simulink model "septum"  (R2024b)
settings: Solver=VariableStepAuto  StartTime=0.0  StopTime=4  RelTol=1e-3
InitFcn:
  | Tint = 1e-6
  | Ts = 100*Tint
libraries: spsIGBTDiodeLib x6, spsSeriesRLCBranchLib x5, spsCurrentMeasurementLib x4, spsVoltageMeasurementLib x4, simulink x2, spsGroundLib x1, spsPowerPositiveSequenceLib x1, spsThreePhaseVIMeasurementLib x1, spsThreePhaseSourceLib x1, spspowerguiLib x1
settings Model: Creator=dagua  LastModifiedBy=dagua
settings DataIOCC: ReturnWorkspaceOutputs=off

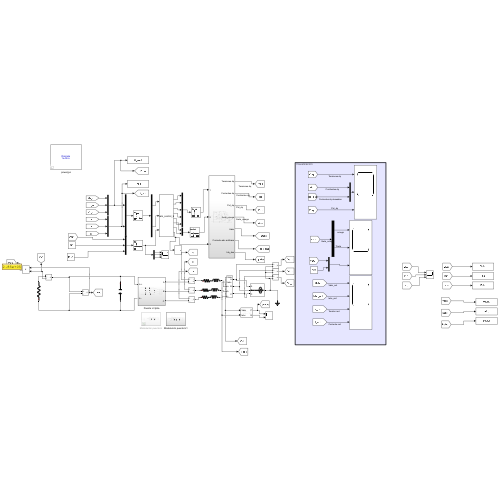
[thumbnail: Simulink's stored preview of the top-level diagram]
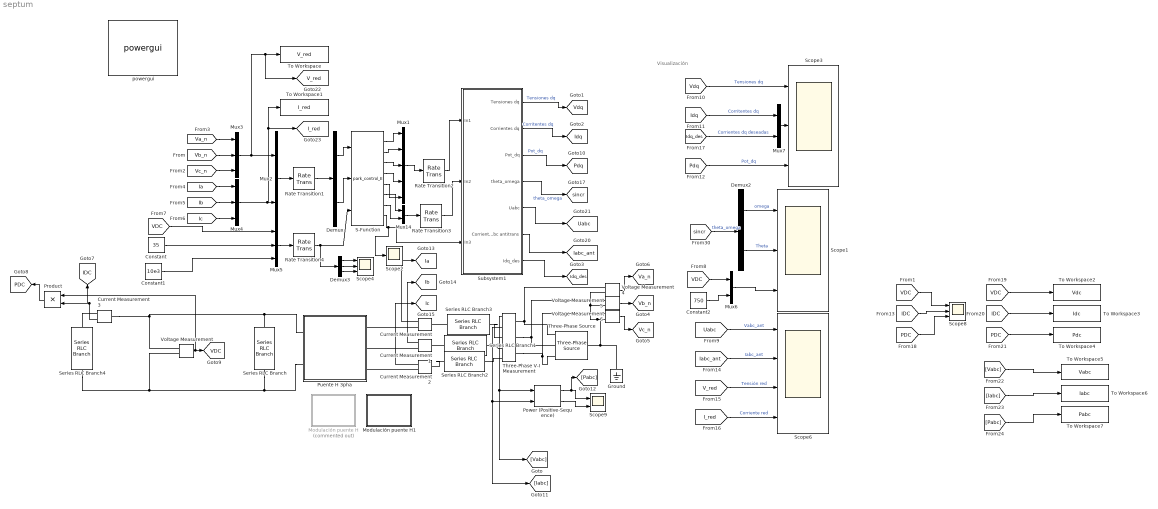
== system septum ==
  note: Visualización
  Constant : Constant  Value=35
  Constant1 : Constant  Value=10e3
  Constant2 : Constant  Value=750
  Current Measurement{,1..3} (4 alike) : spsCurrentMeasurementLib/Current Measurement  PhasorSimulation=off  OutputType=Complex  PSBequivalent=0
  Demux : Demux  Outputs=2
  Demux2 : Demux  Outputs=2
  Demux3 : Demux  Outputs=3
  Ground : spsGroundLib/Ground  LConnTagsString=a
  Modulación puente H : Subsystem  Commented=on
  Modulación puente H1 : Subsystem
  Mux1 : Mux  Inputs=5
  Mux{2,6..7,14} (4 alike) : Mux  Inputs=2
  Mux3 : Mux  Inputs=3
  Mux4 : Mux  Inputs=3
  Mux5 : Mux  Inputs=3
  Power (Positive-Sequence) : spsPowerPositiveSequenceLib/Power (Positive-Sequence)  Freq=50  Vinit=[0, 0]  Iinit=[0, 0]  Ts=0
      settings: LibrarySourceBlock=|
      | sps_lib/Sensors and Measurements/Power
      | (Positive-Sequence)
  Product : Product
  Puente H 3pha : Subsystem
  Rate Transition1 : RateTransition  OutPortSampleTime=Ts
  Rate Transition2 : RateTransition  Deterministic=off  InitialCondition=[0]  OutPortSampleTime=Tint
  Rate Transition3 : RateTransition  Deterministic=off  InitialCondition=[0]  OutPortSampleTime=Tint
  Rate Transition4 : RateTransition  OutPortSampleTime=Ts
  S-Function : S-Function  FunctionName=park_control_E  SFunctionDeploymentMode=off  EnableBusSupport=off
  Scope{1,3..4,8} (4 alike) : Scope  NumInputPorts=3
  Scope2 : Scope
  Scope6 : Scope  NumInputPorts=4
  Scope9 : Scope  NumInputPorts=2
  Series RLC Branch : spsSeriesRLCBranchLib/Series RLC Branch  LConnTagsString=__new0  RConnTagsString=__new0  BranchType=C  Resistance=1  Inductance=1e-3  SetiL0=off  InitialCurrent=0  Capacitance=3300e-4  Setx0=on  InitialVoltage=10  Measurements=None
  Series RLC Branch1 : spsSeriesRLCBranchLib/Series RLC Branch  LConnTagsString=__new0  RConnTagsString=__new0  BranchType=RL  Resistance=0.01  Inductance=12e-5  SetiL0=off  InitialCurrent=0  Capacitance=1e-6  Setx0=off  InitialVoltage=0  Measurements=None
  Series RLC Branch2 : spsSeriesRLCBranchLib/Series RLC Branch  LConnTagsString=__new0  RConnTagsString=__new0  BranchType=RL  Resistance=0.01  Inductance=12e-5  SetiL0=off  InitialCurrent=0  Capacitance=1e-6  Setx0=off  InitialVoltage=0  Measurements=None
  Series RLC Branch3 : spsSeriesRLCBranchLib/Series RLC Branch  LConnTagsString=__new0  RConnTagsString=__new0  BranchType=RL  Resistance=0.01  Inductance=12e-5  SetiL0=off  InitialCurrent=0  Capacitance=1e-6  Setx0=off  InitialVoltage=0  Measurements=None
  Series RLC Branch4 : spsSeriesRLCBranchLib/Series RLC Branch  LConnTagsString=__new0  RConnTagsString=__new0  BranchType=R  Resistance=35*35/267.47e3  Inductance=1e-3  SetiL0=off  InitialCurrent=0  Capacitance=1e-6  Setx0=off  InitialVoltage=0  Measurements=None
  Subsystem1 : Subsystem
  Three-Phase V-I Measurement : spsThreePhaseVIMeasurementLib/Three-Phase V-I Measurement  VoltageMeasurement=phase-to-ground  SetLabelV=off  LabelV=Vabc  Vpu=off  VpuLL=off  CurrentMeasurement=yes  SetLabelI=off  LabelI=Iabc  Ipu=off  Pbase=100e6  Vbase=500e3  OutputType=Complex  PhasorSimulation=off  PSBequivalent=0
  Three-Phase Source : spsThreePhaseSourceLib/Three-Phase Source  InternalConnection=Yn  VoltagePhases=off  Voltage=400  PhaseAngle=0  Voltage_phases=[25e3 25e3 25e3]/sqrt(3)  PhaseAngles_phases=[0 -120 +120]  Frequency=50  NonIdealSource=off  SpecifyImpedance=off  Resistance=0.8929  Inductance=16.58e-3  ShortCircuitLevel=100e6  BaseVoltage=25e3  XRratio=7  BusType=PV  Pref=400e3  Qref=0  Prefabc=[10e3, 10e3, 10e3]  Qrefabc=[0, 0, 0]  Qmin=-inf  Qmax=inf
  To Workspace : ToWorkspace  VariableName=V_red  SaveFormat=Timeseries  SampleTime=-1
  To Workspace1 : ToWorkspace  VariableName=I_red  SaveFormat=Timeseries  SampleTime=-1
  To Workspace2 : ToWorkspace  VariableName=Vdc  SaveFormat=Timeseries  SampleTime=-1
  To Workspace3 : ToWorkspace  VariableName=Idc  SaveFormat=Timeseries  SampleTime=-1
  To Workspace4 : ToWorkspace  VariableName=Pdc  SaveFormat=Timeseries  SampleTime=-1
  To Workspace5 : ToWorkspace  VariableName=Vabc  SaveFormat=Timeseries  SampleTime=-1
  To Workspace6 : ToWorkspace  VariableName=Iabc  SaveFormat=Timeseries  SampleTime=-1
  To Workspace7 : ToWorkspace  VariableName=Pabc  SaveFormat=Timeseries  SampleTime=-1
  Voltage Measurement{,4..6} (4 alike) : spsVoltageMeasurementLib/Voltage Measurement  PhasorSimulation=off  OutputType=Complex  PSBequivalent=0
  powergui : spspowerguiLib/powergui  Priority=1  SimulationMode=Discrete  SampleTime=Tint  frequency=60  Iterations=50  frequencyindice=0  Pbase=100e6  ErrMax=1e-4  UnitsV=kV  UnitsW=MW  buscounter=0  FunctionMessages=off  echomessages=off  EnableUseOfTLC=off  CurrentSourceSwitches=off  DisableSnubberDevices=off  DisableRonSwitches=off  DisableVfSwitches=off  DisplayEquations=off  AutomaticDiscreteSolvers=off  SolverType=Tustin  Interpol=off  ExternalGateDelay=off  methode=off  Ts=0  x0status=blocks  SPID=off  SwTol=0  HookPort=off  NonlinearTolerance=1e-4  nMaxIteration=100  ContinueOnMaxIteration=off  RestoreLinks=warning  ResistiveCurrentMeasurement=off  Frange=[0:2:500]  Ylog=off  Xlog=on  ShowGrid=off  save=off  variable=ZData  structure=Iabc  ZoomFFT=off  StartTime=0.36  cycles=2  DisplayStyle=1  fundamental=50  FreqAxis=off  MaxFrequency=2500  frequencyindicesteady=1  RmsSteady=1  display=off
  tag scope: IDC=global, I_red=global, Ia=global, Iabc_ant=global, Ib=global, Ic=global, Idq=global, Idq_des=global, PDC=global, Pdq=global, Uabc=global, VDC=global, V_red=global, Va_n=global, Vb_n=global, Vc_n=global, Vdq=global, sincr=global
  wires:
  Mux2/1 -> Rate Transition1/1
  S-Function/1 -> Mux1/1
  [Ia] -> Mux4/1
  Rate Transition3/1 -> Subsystem1/2(In2)
  [Ic] -> Mux4/3
  Mux14/1 -> Rate Transition3/1
  Mux3/1 -> [V_red], To Workspace/1, Mux2/1
  Mux5/1 -> Rate Transition4/1
  [V_red] -> Scope6/3  "Tensión red"
  Demux/2 -> S-Function/2
  Demux2/2 -> Scope1/2  "Theta"
  [Pdq] -> Scope3/3  "Pot_dq"
  Subsystem1/7(Idq_des) -> [Idq_des]
  Voltage Measurement/1 -> Product/1, [VDC]
  Current Measurement/1 -> [Ia]
  [VDC] -> Mux6/1
  [Uabc] -> Scope6/1  "Vabc_ant"
  Demux2/1 -> Scope1/1  "omega"
  Demux/1 -> S-Function/1
  [sincr] -> Demux2/1  "theta_omega"
  [Idq] -> Mux7/1  "Corritentes dq"
  [Va_n] -> Mux3/1
  S-Function/6 -> Mux14/1
  Subsystem1/5(Uabc) -> [Uabc]
  S-Function/7 -> Mux14/2
  Subsystem1/1(Tensiones dq) -> [Vdq]  "Tensiones dq"
  Voltage Measurement4/1 -> [Va_n]
  S-Function/5 -> Mux1/5
  [Vdq] -> Scope3/1  "Tensiones dq"
  S-Function/4 -> Mux1/4
  [Ib] -> Mux4/2
  Subsystem1/4(theta_omega) -> [sincr]  "theta_omega"
  Voltage Measurement6/1 -> [Vc_n]
  Subsystem1/2(Corrientes dq) -> [Idq]  "Corritentes dq"
  [Idq_des] -> Mux7/2  "Corrientes dq deseadas"
  [Iabc_ant] -> Scope6/2  "Iabc_ant"
  Rate Transition4/1 -> Demux3/1, S-Function/3
  Mux4/1 -> To Workspace1/1, [I_red], Mux2/2
  Current Measurement2/1 -> [Ic]
  Constant2/1 -> Mux6/2
  Mux1/1 -> Rate Transition2/1
  Subsystem1/6(Corriente abc antitrans) -> [Iabc_ant]
  S-Function/2 -> Mux1/2
  [VDC] -> Mux5/1
  Voltage Measurement5/1 -> [Vb_n]
  S-Function/3 -> Mux1/3
  Rate Transition2/1 -> Subsystem1/1(In1)
  [Vc_n] -> Mux3/3
  [I_red] -> Scope6/4  "Corriente red"
  Current Measurement1/1 -> [Ib]
  Mux7/1 -> Scope3/2
  Constant/1 -> Mux5/2
  Constant1/1 -> Mux5/3
  [Vb_n] -> Mux3/2
  Subsystem1/3(Pot_dq) -> [Pdq]  "Pot_dq"
  Rate Transition1/1 -> Demux/1
  Mux6/1 -> Scope1/3
  Current Measurement3/1 -> [IDC], Product/2
  Product/1 -> [PDC]
  Demux3/1 -> Scope4/1
  Demux3/2 -> Scope4/2
  Demux3/3 -> Scope4/3
  S-Function/8 -> Scope2/1, Subsystem1/3(In3)
  [Pabc] -> To Workspace7/1
  [IDC] -> Scope8/2
  [PDC] -> Scope8/3
  [VDC] -> To Workspace2/1
  [PDC] -> To Workspace4/1
  [VDC] -> Scope8/1
  [Iabc] -> To Workspace6/1
  [IDC] -> To Workspace3/1
  [Vabc] -> To Workspace5/1
  Power (Positive-Sequence)/1 -> [Pabc], Scope9/1
  Power (Positive-Sequence)/2 -> Scope9/2
  Three-Phase V-I Measurement/2 -> [Iabc], Power (Positive-Sequence)/2
  Three-Phase V-I Measurement/1 -> Power (Positive-Sequence)/1, [Vabc]
  connections:
  Voltage Measurement4/LConn2 -- Voltage Measurement5/LConn2 -- Voltage Measurement6/LConn2 -- Three-Phase Source/LConn1 -- Ground/LConn1
  Puente H 3pha/LConn1 -- Current Measurement3/LConn1 -- Voltage Measurement/LConn1 -- Series RLC Branch/LConn1
  Three-Phase Source/RConn3 -- Three-Phase V-I Measurement/LConn3 -- Voltage Measurement6/LConn1
  Puente H 3pha/LConn2 -- Series RLC Branch4/LConn1 -- Voltage Measurement/LConn2 -- Series RLC Branch/RConn1
  Voltage Measurement4/LConn1 -- Three-Phase V-I Measurement/LConn1 -- Three-Phase Source/RConn1
  Three-Phase Source/RConn2 -- Three-Phase V-I Measurement/LConn2 -- Voltage Measurement5/LConn1
  Current Measurement/RConn1 -- Puente H 3pha/RConn1
  Current Measurement2/RConn1 -- Puente H 3pha/RConn3
  Series RLC Branch1/LConn1 -- Current Measurement1/LConn1
  Series RLC Branch2/LConn1 -- Current Measurement2/LConn1
  Series RLC Branch3/LConn1 -- Current Measurement/LConn1
  Current Measurement1/RConn1 -- Puente H 3pha/RConn2
  Series RLC Branch4/RConn1 -- Current Measurement3/RConn1
  Series RLC Branch3/RConn1 -- Three-Phase V-I Measurement/RConn1
  Series RLC Branch1/RConn1 -- Three-Phase V-I Measurement/RConn2
  Series RLC Branch2/RConn1 -- Three-Phase V-I Measurement/RConn3

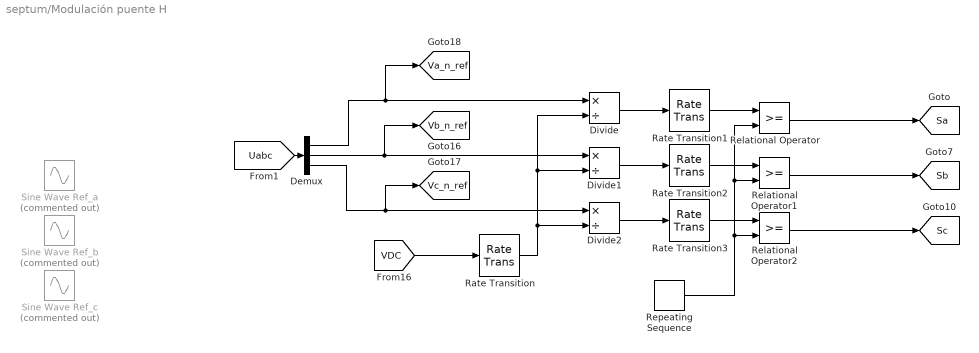
== system septum/Modulación puente H ==
  Demux : Demux  Outputs=3
  Divide : Product  Inputs=*/
  Divide1 : Product  Inputs=*/
  Divide2 : Product  Inputs=*/
  Rate Transition : RateTransition  OutPortSampleTime=Ts
  Rate Transition1 : RateTransition  OutPortSampleTime=Tint
  Rate Transition2 : RateTransition  OutPortSampleTime=Tint
  Rate Transition3 : RateTransition  OutPortSampleTime=Tint
  Relational Operator : RelationalOperator  OutDataTypeStr=boolean  RndMeth=Simplest  InputSameDT=off
  Relational Operator1 : RelationalOperator  OutDataTypeStr=boolean  RndMeth=Simplest  InputSameDT=off
  Relational Operator2 : RelationalOperator  OutDataTypeStr=boolean  RndMeth=Simplest  InputSameDT=off
  Repeating Sequence : simulink/Sources/Repeating Sequence  rep_seq_t=[0 Ts/2 Ts]  rep_seq_y=[-1 1 -1]
  Sine Wave Ref_a : Sin  Commented=on  Amplitude=370  Frequency=2*pi*50  SampleTime=Ts
  Sine Wave Ref_b : Sin  Commented=on  Amplitude=370  Frequency=2*pi*50  Phase=120*2*pi/360  SampleTime=Ts
  Sine Wave Ref_c : Sin  Commented=on  Amplitude=370  Frequency=2*pi*50  Phase=-120*2*pi/360  SampleTime=Ts
  tag scope: Sa=global, Sb=global, Sc=global, Va_n_ref=global, Vb_n_ref=global, Vc_n_ref=global
  wires:
  Demux/3 -> [Vc_n_ref], Divide2/1
  Demux/1 -> Divide/1, [Va_n_ref]
  Demux/2 -> [Vb_n_ref], Divide1/1
  [VDC] -> Rate Transition/1
  Relational Operator/1 -> [Sa]
  Relational Operator1/1 -> [Sb]
  Relational Operator2/1 -> [Sc]
  Rate Transition/1 -> Divide2/2, Divide1/2, Divide/2
  Rate Transition1/1 -> Relational Operator/1
  Divide1/1 -> Rate Transition2/1
  Rate Transition2/1 -> Relational Operator1/1
  Divide2/1 -> Rate Transition3/1
  Rate Transition3/1 -> Relational Operator2/1
  Repeating Sequence/1 -> Relational Operator2/2, Relational Operator1/2, Relational Operator/2
  Divide/1 -> Rate Transition1/1
  [Uabc] -> Demux/1

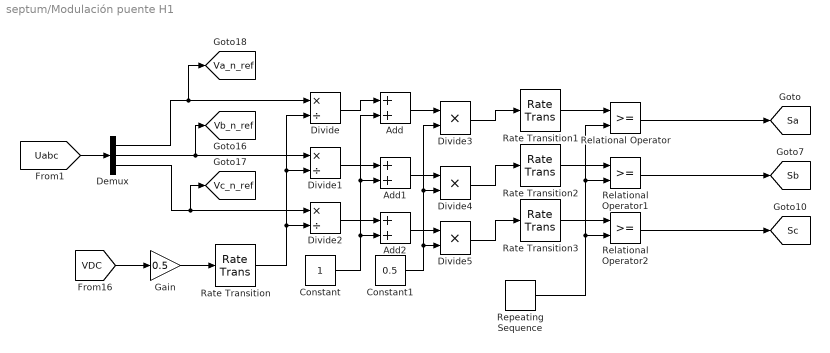
== system septum/Modulación puente H1 ==
  Add : Sum
  Add1 : Sum
  Add2 : Sum
  Constant : Constant
  Constant1 : Constant  Value=0.5
  Demux : Demux  Outputs=3
  Divide : Product  Inputs=*/
  Divide1 : Product  Inputs=*/
  Divide2 : Product  Inputs=*/
  Divide3 : Product  Inputs=**
  Divide4 : Product  Inputs=**
  Divide5 : Product  Inputs=**
  Gain : Gain  Gain=0.5
  Rate Transition : RateTransition  OutPortSampleTime=Ts
  Rate Transition1 : RateTransition  OutPortSampleTime=Tint
  Rate Transition2 : RateTransition  OutPortSampleTime=Tint
  Rate Transition3 : RateTransition  OutPortSampleTime=Tint
  Relational Operator : RelationalOperator  OutDataTypeStr=boolean  RndMeth=Simplest  InputSameDT=off
  Relational Operator1 : RelationalOperator  OutDataTypeStr=boolean  RndMeth=Simplest  InputSameDT=off
  Relational Operator2 : RelationalOperator  OutDataTypeStr=boolean  RndMeth=Simplest  InputSameDT=off
  Repeating Sequence : simulink/Sources/Repeating Sequence  rep_seq_t=[0 Ts/2 Ts]  rep_seq_y=[0 1 0]
  tag scope: Sa=global, Sb=global, Sc=global, Va_n_ref=global, Vb_n_ref=global, Vc_n_ref=global
  wires:
  Demux/3 -> [Vc_n_ref], Divide2/1
  Demux/1 -> [Va_n_ref], Divide/1
  Demux/2 -> [Vb_n_ref], Divide1/1
  [VDC] -> Gain/1
  Relational Operator/1 -> [Sa]
  Relational Operator1/1 -> [Sb]
  Relational Operator2/1 -> [Sc]
  Rate Transition/1 -> Divide1/2, Divide/2, Divide2/2
  Rate Transition1/1 -> Relational Operator/1
  Rate Transition2/1 -> Relational Operator1/1
  Rate Transition3/1 -> Relational Operator2/1
  Repeating Sequence/1 -> Relational Operator2/2, Relational Operator1/2, Relational Operator/2
  Divide/1 -> Add/1
  Add/1 -> Divide3/1
  Divide3/1 -> Rate Transition1/1
  Add1/1 -> Divide4/1
  Add2/1 -> Divide5/1
  Divide1/1 -> Add1/1
  Divide4/1 -> Rate Transition2/1
  Divide2/1 -> Add2/1
  Divide5/1 -> Rate Transition3/1
  Constant/1 -> Add2/2, Add1/2, Add/2
  Constant1/1 -> Divide5/2, Divide4/2, Divide3/2
  [Uabc] -> Demux/1
  Gain/1 -> Rate Transition/1

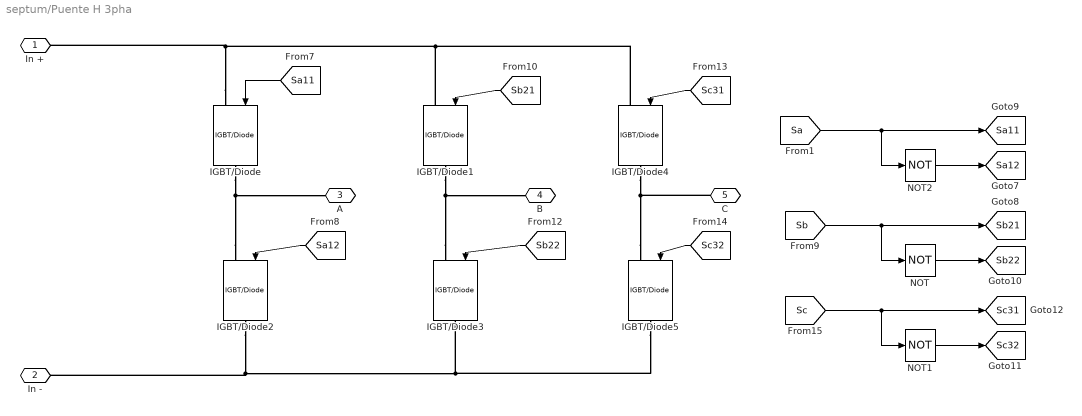
== system septum/Puente H 3pha ==
  IGBT/Diode{,1..5} (6 alike) : spsIGBTDiodeLib/IGBT//Diode  Ron=1e-3  Rs=1e5  Cs=inf  Measurements=off
  NOT : Logic  Operator=NOT  IconShape=distinctive  AllPortsSameDT=off  OutDataTypeStr=boolean
  NOT1 : Logic  Operator=NOT  IconShape=distinctive  AllPortsSameDT=off  OutDataTypeStr=boolean
  NOT2 : Logic  Operator=NOT  IconShape=distinctive  AllPortsSameDT=off  OutDataTypeStr=boolean
  In + : PMIOPort  Side=Left
  In - : PMIOPort  Port=2  Side=Left
  A : PMIOPort  Port=3  Side=Right
  B : PMIOPort  Port=4  Side=Right
  C : PMIOPort  Port=5  Side=Right
  tag scope: Sa11=global, Sa12=global, Sb21=global, Sb22=global, Sc31=global, Sc32=global
  wires:
  [Sa11] -> IGBT/Diode/1
  [Sc31] -> IGBT/Diode4/1
  [Sb] -> [Sb21], NOT/1
  [Sc32] -> IGBT/Diode5/1
  NOT2/1 -> [Sa12]
  NOT/1 -> [Sb22]
  [Sa] -> [Sa11], NOT2/1
  [Sb21] -> IGBT/Diode1/1
  [Sa12] -> IGBT/Diode2/1
  [Sb22] -> IGBT/Diode3/1
  NOT1/1 -> [Sc32]
  [Sc] -> [Sc31], NOT1/1
  connections:
  IGBT/Diode2/LConn1 -- A/RConn1 -- IGBT/Diode/RConn1
  IGBT/Diode5/LConn1 -- C/RConn1 -- IGBT/Diode4/RConn1
  In -/RConn1 -- IGBT/Diode2/RConn1 -- IGBT/Diode5/RConn1 -- IGBT/Diode3/RConn1
  IGBT/Diode/LConn1 -- In +/RConn1 -- IGBT/Diode4/LConn1 -- IGBT/Diode1/LConn1
  IGBT/Diode3/LConn1 -- B/RConn1 -- IGBT/Diode1/RConn1

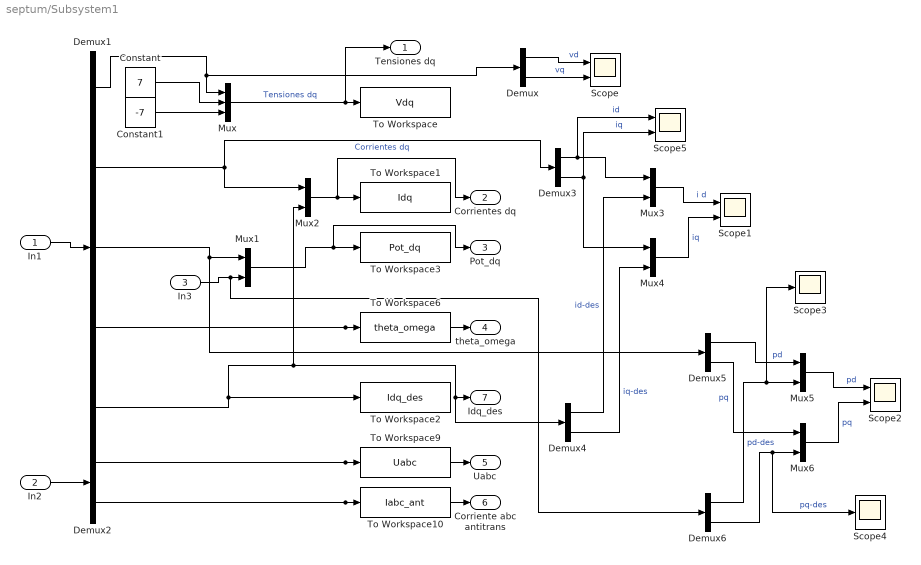
== system septum/Subsystem1 ==
  In1 : Inport
  In2 : Inport  Port=2
  In3 : Inport  Port=3
  Constant : Constant  Value=7
  Constant1 : Constant  Value=-7
  Demux{,2..6} (6 alike) : Demux  Outputs=2
  Demux1 : Demux  Outputs=5
  Mux : Mux  Inputs=3
  Mux{1..6} (6 alike) : Mux  Inputs=2
  Scope{,1..2,5} (4 alike) : Scope  NumInputPorts=2
  Scope3 : Scope
  Scope4 : Scope
  To Workspace : ToWorkspace  VariableName=Vdq  SaveFormat=Timeseries  SampleTime=-1
  To Workspace1 : ToWorkspace  VariableName=Idq  SaveFormat=Timeseries  SampleTime=-1
  To Workspace10 : ToWorkspace  VariableName=Iabc_ant  SaveFormat=Timeseries  SampleTime=-1
  To Workspace2 : ToWorkspace  VariableName=Idq_des  SaveFormat=Timeseries  SampleTime=-1
  To Workspace3 : ToWorkspace  VariableName=Pot_dq  SaveFormat=Timeseries  SampleTime=-1
  To Workspace6 : ToWorkspace  VariableName=theta_omega  SaveFormat=Timeseries  SampleTime=-1
  To Workspace9 : ToWorkspace  VariableName=Uabc  SaveFormat=Timeseries  SampleTime=-1
  Tensiones dq : Outport
  Corrientes dq : Outport  Port=2
  Pot_dq : Outport  Port=3
  theta_omega : Outport  Port=4
  Uabc : Outport  Port=5
  Corriente abc antitrans : Outport  Port=6
  Idq_des : Outport  Port=7
  wires:
  Mux/1 -> Tensiones dq/1, To Workspace/1  "Tensiones dq"
  Constant1/1 -> Mux/3
  Constant/1 -> Mux/2
  Demux1/1 -> Mux/1, Demux/1
  In1/1 -> Demux1/1
  Demux2/1 -> Uabc/1, To Workspace9/1
  Demux2/2 -> Corriente abc antitrans/1, To Workspace10/1
  In2/1 -> Demux2/1
  Demux1/4 -> theta_omega/1, To Workspace6/1
  Demux1/5 -> To Workspace2/1, Mux2/2, Demux4/1, Idq_des/1
  Demux1/3 -> Demux5/1, Mux1/1
  In3/1 -> Demux6/1, Mux1/2
  Mux1/1 -> Pot_dq/1, To Workspace3/1
  Demux1/2 -> Mux2/1, Demux3/1  "Corrientes dq"
  Mux2/1 -> Corrientes dq/1, To Workspace1/1
  Demux/1 -> Scope/1  "vd"
  Demux/2 -> Scope/2  "vq"
  Demux3/1 -> Scope5/1, Mux3/1  "id"
  Demux3/2 -> Mux4/1, Scope5/2  "iq"
  Demux4/1 -> Mux3/2  "id-des"
  Demux4/2 -> Mux4/2  "iq-des"
  Mux3/1 -> Scope1/1  "i d"
  Mux4/1 -> Scope1/2  "iq"
  Demux5/2 -> Mux6/1  "pq"
  Demux6/1 -> Scope3/1, Mux5/2  "pd-des"
  Demux6/2 -> Scope4/1, Mux6/2  "pq-des"
  Mux5/1 -> Scope2/1  "pd"
  Demux5/1 -> Mux5/1  "pd"
  Mux6/1 -> Scope2/2  "pq"
